simulink model "FaceDet_x4"  (Simulink 7.7)
settings: Solver=FixedStepDiscrete  StartTime=0  StopTime=10  RelTol=1e-3
libraries: simulink x257
(part 1 of 5)
settings Model: Creator=Ilia  LastModifiedBy=iliav
settings OptimizationCC: BlockReduction=off  ConditionallyExecuteInputs=off
settings DebuggingCC: StrictBusMsg=Warning

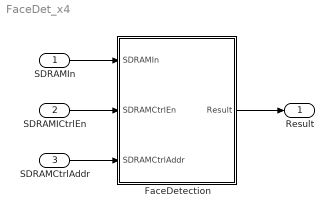
== system FaceDet_x4 ==
  SDRAMIn : Inport  OutDataTypeStr=uint(5)
  SDRAMICtrlEn : Inport  Port=2  OutDataTypeStr=boolean
  SDRAMCtrlAddr : Inport  Port=3  OutDataTypeStr=uint(12)
  FaceDetection : Subsystem
  Result : Outport
  wires:
  FaceDetection/1(Result) -> Result/1
  SDRAMIn/1 -> FaceDetection/1(SDRAMIn)
  SDRAMICtrlEn/1 -> FaceDetection/2(SDRAMCtrlEn)
  SDRAMCtrlAddr/1 -> FaceDetection/3(SDRAMCtrlAddr)

== system FaceDet_x4/FaceDetection ==
  SDRAMIn : Inport
  SDRAMCtrlEn : Inport  Port=2
  SDRAMCtrlAddr : Inport  Port=3
  DU : Subsystem
      mask Display: disp( 'Delay Lines\nUnit\n' )
  FU : Subsystem
      mask Display: disp( 'Face Detection\nUnit' )
  Result : Outport
  wires:
  DU/1(DOut24x5) -> FU/1(DIn24x5)
  SDRAMIn/1 -> DU/3(Data)
  SDRAMCtrlEn/1 -> DU/2(DLCtrlEn)
  SDRAMCtrlAddr/1 -> DU/1(DLCtrlAdr)
  FU/1(Result) -> Result/1

== system FaceDet_x4/FaceDetection/DU ==
  DLCtrlAdr : Inport
  DLCtrlEn : Inport  Port=2
  Data : Inport  Port=3
  Comb24DL : Mux  Inputs=3
  SplittedDL1 : Subsystem  TreatAsAtomicUnit=on
      mask Display: disp( 'Splitted DL\n8x512x5' )
  SplittedDL2 : Subsystem  TreatAsAtomicUnit=on
      mask Display: disp( 'Splitted DL\n8x512x5' )
  SplittedDL3 : Subsystem  TreatAsAtomicUnit=on
      mask Display: disp( 'Splitted DL\n8x512x5' )
  DOut24x5 : Outport
  wires:
  DLCtrlAdr/1 -> SplittedDL2/1(WrAdr), SplittedDL1/1(WrAdr), SplittedDL3/1(WrAdr), SplittedDL2/2(RdAdr), SplittedDL1/2(RdAdr), SplittedDL3/2(RdAdr)
  Comb24DL/1 -> DOut24x5/1
  SplittedDL3/1(DOut8x5) -> Comb24DL/1
  SplittedDL1/1(DOut8x5) -> Comb24DL/3
  SplittedDL2/1(DOut8x5) -> Comb24DL/2
  DLCtrlEn/1 -> SplittedDL2/3(WrEn), SplittedDL1/3(WrEn), SplittedDL3/3(WrEn)
  Data/1 -> SplittedDL3/4(DIn1x5), SplittedDL2/4(DIn1x5), SplittedDL1/4(DIn1x5)

== system FaceDet_x4/FaceDetection/FU ==
  DIn24x5 : Inport
  AccumulateAllFeatures : Subsystem  TreatAsAtomicUnit=on  mask(Accumulator){NBits=18}
      mask prompts: NBits "Number of Bits"
      mask help:
      | Accumulates incoming data. On reset only the state is initialized, meaning that when the reset is asserted the first valid output will be available from the next clock.
      | It is user responsiblity not to overcome the capacity of the accumulator.
      mask Help: web( ['E:\Ilia\Sightic\MakeVerilog\AccBlk\', 'AccBlkHelp.htm'] )
      mask Display: disp( 'Acc Blk\nBDelay = 0' )
  AddAllFeatures : Sum  Inputs=++++  OutDataTypeStr=uint(18)
  CalcIntegralImg : Subsystem  RequirementInfo={} %GIDa_13edc57c_8db7_4be7_a667_2f88c1a358e2  TreatAsAtomicUnit=on
  CalcNNVariance : Subsystem  TreatAsAtomicUnit=on
  CompToStrongTresh : RelationalOperator  Operator=<  OutDataTypeStr=boolean
  Demux1 : Demux
  Demux2 : Demux
  FaceDetectionControl : Stateflow chart  TreatAsAtomicUnit=on
      settings: RTWSystemCode=Inline
  FeatureCalcMachine0 : Subsystem  TreatAsAtomicUnit=on
      mask Display: disp( 'BDelay = \n' )
  FeatureCalcMachine1 : Subsystem  TreatAsAtomicUnit=on
      mask Display: disp( 'BDelay = \n' )
  FeatureCalcMachine2 : Subsystem  TreatAsAtomicUnit=on
      mask Display: disp( 'BDelay = \n' )
  FeatureCalcMachine3 : Subsystem  TreatAsAtomicUnit=on
      mask Display: disp( 'BDelay = \n' )
  MemBank : Subsystem
      mask Display: disp( '            Memory Block\n\n' )
  ValidNNTerm : Terminator
  Result : Outport
  wires:
  DIn24x5/1 -> CalcIntegralImg/1(DIn24x5), CalcNNVariance/2(Lines24x15)
  CalcIntegralImg/3(DOut24x15) -> FeatureCalcMachine2/2(Lines24x15), FeatureCalcMachine3/2(Lines24x15), FeatureCalcMachine1/2(Lines24x15), FeatureCalcMachine0/2(Lines24x15)
  MemBank/1(LineIdxs) -> FeatureCalcMachine2/3(LineIdxs), FeatureCalcMachine3/3(LineIdxs), FeatureCalcMachine1/3(LineIdxs), FeatureCalcMachine0/3(LineIdxs)
  MemBank/2(NodeWeights) -> FeatureCalcMachine2/4(NodeWeights), FeatureCalcMachine3/4(NodeWeights), FeatureCalcMachine1/4(NodeWeights), FeatureCalcMachine0/4(NodeWeights)
  FeatureCalcMachine0/1(FinalFeatureWeight) -> AddAllFeatures/1
  MemBank/4(StrongTresh) -> CompToStrongTresh/1
  CompToStrongTresh/1 -> Result/1
  AddAllFeatures/1 -> AccumulateAllFeatures/1(In)
  MemBank/3(FeatureData) -> Demux1/1
  Demux1/1 -> FeatureCalcMachine0/5(FeatureData)
  MemBank/5(WeakTresh) -> Demux2/1
  Demux2/1 -> FeatureCalcMachine0/6(WeakTresh)
  FeatureCalcMachine1/1(FinalFeatureWeight) -> AddAllFeatures/2
  FeatureCalcMachine2/1(FinalFeatureWeight) -> AddAllFeatures/3
  Demux1/2 -> FeatureCalcMachine1/5(FeatureData)
  AccumulateAllFeatures/1(Acc) -> CompToStrongTresh/2
  Demux1/3 -> FeatureCalcMachine2/5(FeatureData)
  Demux2/2 -> FeatureCalcMachine1/6(WeakTresh)
  Demux2/3 -> FeatureCalcMachine2/6(WeakTresh)
  FeatureCalcMachine3/1(FinalFeatureWeight) -> AddAllFeatures/4
  Demux1/4 -> FeatureCalcMachine3/5(FeatureData)
  Demux2/4 -> FeatureCalcMachine3/6(WeakTresh)
  CalcNNVariance/1(SqVar) -> FeatureCalcMachine2/1(SqVar), FeatureCalcMachine3/1(SqVar), FeatureCalcMachine1/1(SqVar), FeatureCalcMachine0/1(SqVar)
  CalcIntegralImg/1(MeanBlkVal) -> CalcNNVariance/3(MeanBlkVal)
  CalcIntegralImg/2(ValidNN) -> ValidNNTerm/1
  FaceDetectionControl/3(LatchIdxLatch) -> MemBank/1(LineIdxsLatch)
  FaceDetectionControl/4(LatchIdxExt) -> MemBank/2(LineIdxsExt)
  FaceDetectionControl/5(NodeWeightsCtrlRdAdr) -> MemBank/3(NodeWeightsCtrlRdAdr)
  FaceDetectionControl/6(NodeWeightsCtrlWrAdr) -> MemBank/4(NodeWeightsCtrlWrAdr)
  FaceDetectionControl/7(NodeWeightsCtrlEn) -> MemBank/5(NodeWeightsCtrlEn)
  FaceDetectionControl/8(NodeWeightsExt) -> MemBank/6(NodeWeightsExt)
  FaceDetectionControl/9(FeatureDataLatch) -> MemBank/7(FeatureDataLatch)
  FaceDetectionControl/10(FeatureDataExt) -> MemBank/8(FeatureDataExt)
  FaceDetectionControl/11(WeakTreshLatch) -> MemBank/9(WeakTreshLatch)
  FaceDetectionControl/12(WeakTreshExt) -> MemBank/10(WeakTreshExt)
  FaceDetectionControl/13(StrongTreshLatch) -> MemBank/11(StrongTreshLatch)
  FaceDetectionControl/14(StrongTreshExt) -> MemBank/12(StrongTreshExt)
  FaceDetectionControl/2(Rst) -> CalcIntegralImg/2(Rst), CalcNNVariance/1(Rst), AccumulateAllFeatures/3(Rst)
  FaceDetectionControl/1(En) -> CalcIntegralImg/3(En), AccumulateAllFeatures/2(En)

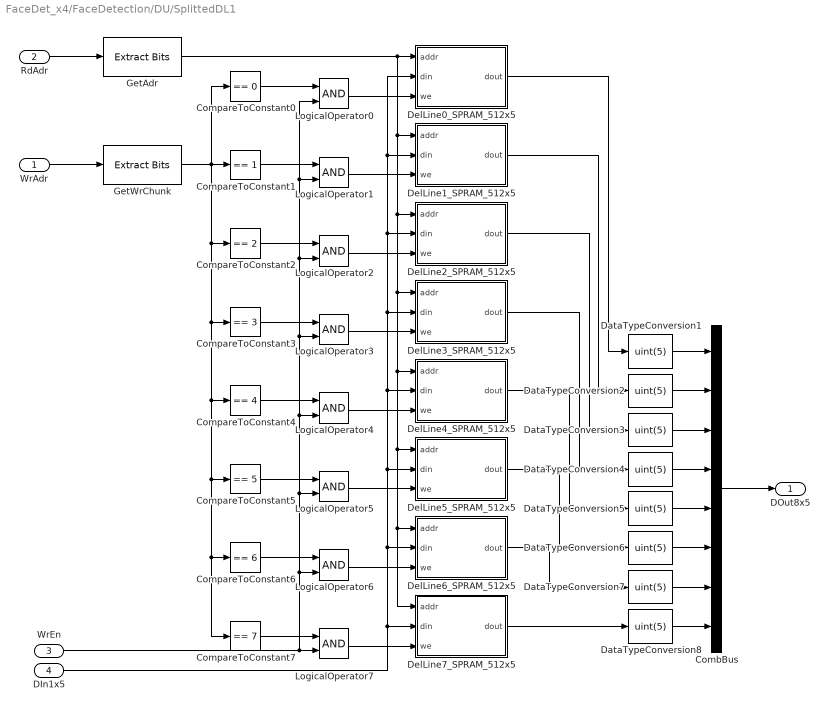
== system FaceDet_x4/FaceDetection/DU/SplittedDL1 ==
  WrAdr : Inport
  RdAdr : Inport  Port=2
  WrEn : Inport  Port=3
  DIn1x5 : Inport  Port=4
  CombBus : Mux  Inputs=8
  CompareToConstant0 : simulink/Logic and Bit Operations/Compare To Constant  SystemSampleTime=-1  relop===  const=0  LogicOutDataTypeMode=boolean  ZeroCross=off
  CompareToConstant1 : simulink/Logic and Bit Operations/Compare To Constant  SystemSampleTime=-1  relop===  const=1  LogicOutDataTypeMode=boolean  ZeroCross=off
  CompareToConstant2 : simulink/Logic and Bit Operations/Compare To Constant  SystemSampleTime=-1  relop===  const=2  LogicOutDataTypeMode=boolean  ZeroCross=off
  CompareToConstant3 : simulink/Logic and Bit Operations/Compare To Constant  SystemSampleTime=-1  relop===  const=3  LogicOutDataTypeMode=boolean  ZeroCross=off
  CompareToConstant4 : simulink/Logic and Bit Operations/Compare To Constant  SystemSampleTime=-1  relop===  const=4  LogicOutDataTypeMode=boolean  ZeroCross=off
  CompareToConstant5 : simulink/Logic and Bit Operations/Compare To Constant  SystemSampleTime=-1  relop===  const=5  LogicOutDataTypeMode=boolean  ZeroCross=off
  CompareToConstant6 : simulink/Logic and Bit Operations/Compare To Constant  SystemSampleTime=-1  relop===  const=6  LogicOutDataTypeMode=boolean  ZeroCross=off
  CompareToConstant7 : simulink/Logic and Bit Operations/Compare To Constant  SystemSampleTime=-1  relop===  const=7  LogicOutDataTypeMode=boolean  ZeroCross=off
  DataTypeConversion{1..8} (8 alike) : DataTypeConversion  OutDataTypeStr=uint(5)
  DelLine0_SPRAM_512x5 : Subsystem  TreatAsAtomicUnit=on  mask(Single-port RAM){BlkNamePrefix='DelLine0', depth_bits=9, width_bits=5, dout_type=New data}
      mask prompts: BlkNamePrefix "Block name prefix:"; depth_bits "Address port width (2 to 16):"; width_bits "Data port width:"; dout_type "Output data during write:"
      mask help:
      | This block simulates a single-port RAM (based on hdllib).
      |
      | The address port width is limited to between 2 to 16 bits.
      mask init:
      | dout_type = 1;
      | 
      | if (isempty(depth_bits) || isempty(width_bits))
      |     set_param(gcb, 'Name', 'Single Port RAM');
      | else
      |     
      |     ram_elements = 2^depth_bits;
      |     
      |     NewName = ['SPRAM_', int2str(ram_elements), ...
      |         'x', int2str(width_bits)];
      |     
      |     if ~isempty(BlkNamePrefix)
      |         NewName = [BlkNamePrefix, '_', NewName];
      |     end
      |     
      |     set_param(gcb, 'Name', NewName);
      | 
      | end
      mask StyleString: edit,edit,edit,popup(New data|Old data)
      mask Display: color('gray'); text(.5, .05, '{\fontsize{6}BRCM}', 'texmode', 'on', 'verticalAlignment', 'bottom', 'horizontalAlignment', 'center');
  DelLine1_SPRAM_512x5 : Subsystem  TreatAsAtomicUnit=on  mask(Single-port RAM){BlkNamePrefix='DelLine1', depth_bits=9, width_bits=5, dout_type=New data}
      mask prompts: BlkNamePrefix "Block name prefix:"; depth_bits "Address port width (2 to 16):"; width_bits "Data port width:"; dout_type "Output data during write:"
      mask help:
      | This block simulates a single-port RAM (based on hdllib).
      |
      | The address port width is limited to between 2 to 16 bits.
      mask init: same as FaceDet_x4/FaceDetection/DU/SplittedDL1/DelLine0_SPRAM_512x5
      mask StyleString: edit,edit,edit,popup(New data|Old data)
      mask Display: color('gray'); text(.5, .05, '{\fontsize{6}BRCM}', 'texmode', 'on', 'verticalAlignment', 'bottom', 'horizontalAlignment', 'center');
  DelLine2_SPRAM_512x5 : Subsystem  TreatAsAtomicUnit=on  mask(Single-port RAM){BlkNamePrefix='DelLine2', depth_bits=9, width_bits=5, dout_type=New data}
      mask prompts: BlkNamePrefix "Block name prefix:"; depth_bits "Address port width (2 to 16):"; width_bits "Data port width:"; dout_type "Output data during write:"
      mask help:
      | This block simulates a single-port RAM (based on hdllib).
      |
      | The address port width is limited to between 2 to 16 bits.
      mask init: same as FaceDet_x4/FaceDetection/DU/SplittedDL1/DelLine0_SPRAM_512x5
      mask StyleString: edit,edit,edit,popup(New data|Old data)
      mask Display: color('gray'); text(.5, .05, '{\fontsize{6}BRCM}', 'texmode', 'on', 'verticalAlignment', 'bottom', 'horizontalAlignment', 'center');
  DelLine3_SPRAM_512x5 : Subsystem  TreatAsAtomicUnit=on  mask(Single-port RAM){BlkNamePrefix='DelLine3', depth_bits=9, width_bits=5, dout_type=New data}
      mask prompts: BlkNamePrefix "Block name prefix:"; depth_bits "Address port width (2 to 16):"; width_bits "Data port width:"; dout_type "Output data during write:"
      mask help:
      | This block simulates a single-port RAM (based on hdllib).
      |
      | The address port width is limited to between 2 to 16 bits.
      mask init: same as FaceDet_x4/FaceDetection/DU/SplittedDL1/DelLine0_SPRAM_512x5
      mask StyleString: edit,edit,edit,popup(New data|Old data)
      mask Display: color('gray'); text(.5, .05, '{\fontsize{6}BRCM}', 'texmode', 'on', 'verticalAlignment', 'bottom', 'horizontalAlignment', 'center');
  DelLine4_SPRAM_512x5 : Subsystem  TreatAsAtomicUnit=on  mask(Single-port RAM){BlkNamePrefix='DelLine4', depth_bits=9, width_bits=5, dout_type=New data}
      mask prompts: BlkNamePrefix "Block name prefix:"; depth_bits "Address port width (2 to 16):"; width_bits "Data port width:"; dout_type "Output data during write:"
      mask help:
      | This block simulates a single-port RAM (based on hdllib).
      |
      | The address port width is limited to between 2 to 16 bits.
      mask init: same as FaceDet_x4/FaceDetection/DU/SplittedDL1/DelLine0_SPRAM_512x5
      mask StyleString: edit,edit,edit,popup(New data|Old data)
      mask Display: color('gray'); text(.5, .05, '{\fontsize{6}BRCM}', 'texmode', 'on', 'verticalAlignment', 'bottom', 'horizontalAlignment', 'center');
  DelLine5_SPRAM_512x5 : Subsystem  TreatAsAtomicUnit=on  mask(Single-port RAM){BlkNamePrefix='DelLine5', depth_bits=9, width_bits=5, dout_type=New data}
      mask prompts: BlkNamePrefix "Block name prefix:"; depth_bits "Address port width (2 to 16):"; width_bits "Data port width:"; dout_type "Output data during write:"
      mask help:
      | This block simulates a single-port RAM (based on hdllib).
      |
      | The address port width is limited to between 2 to 16 bits.
      mask init: same as FaceDet_x4/FaceDetection/DU/SplittedDL1/DelLine0_SPRAM_512x5
      mask StyleString: edit,edit,edit,popup(New data|Old data)
      mask Display: color('gray'); text(.5, .05, '{\fontsize{6}BRCM}', 'texmode', 'on', 'verticalAlignment', 'bottom', 'horizontalAlignment', 'center');
  DelLine6_SPRAM_512x5 : Subsystem  TreatAsAtomicUnit=on  mask(Single-port RAM){BlkNamePrefix='DelLine6', depth_bits=9, width_bits=5, dout_type=New data}
      mask prompts: BlkNamePrefix "Block name prefix:"; depth_bits "Address port width (2 to 16):"; width_bits "Data port width:"; dout_type "Output data during write:"
      mask help:
      | This block simulates a single-port RAM (based on hdllib).
      |
      | The address port width is limited to between 2 to 16 bits.
      mask init: same as FaceDet_x4/FaceDetection/DU/SplittedDL1/DelLine0_SPRAM_512x5
      mask StyleString: edit,edit,edit,popup(New data|Old data)
      mask Display: color('gray'); text(.5, .05, '{\fontsize{6}BRCM}', 'texmode', 'on', 'verticalAlignment', 'bottom', 'horizontalAlignment', 'center');
  DelLine7_SPRAM_512x5 : Subsystem  TreatAsAtomicUnit=on  mask(Single-port RAM){BlkNamePrefix='DelLine7', depth_bits=9, width_bits=5, dout_type=New data}
      mask prompts: BlkNamePrefix "Block name prefix:"; depth_bits "Address port width (2 to 16):"; width_bits "Data port width:"; dout_type "Output data during write:"
      mask help:
      | This block simulates a single-port RAM (based on hdllib).
      |
      | The address port width is limited to between 2 to 16 bits.
      mask init: same as FaceDet_x4/FaceDetection/DU/SplittedDL1/DelLine0_SPRAM_512x5
      mask StyleString: edit,edit,edit,popup(New data|Old data)
      mask Display: color('gray'); text(.5, .05, '{\fontsize{6}BRCM}', 'texmode', 'on', 'verticalAlignment', 'bottom', 'horizontalAlignment', 'center');
  GetAdr : simulink/Logic and Bit Operations/Extract Bits  SystemSampleTime=-1  bitsToExtract=Range of bits  numBits=8  bitIdxRange=[0 8]  outScalingMode=Treat bit field as an integer
  GetWrChunk : simulink/Logic and Bit Operations/Extract Bits  SystemSampleTime=-1  bitsToExtract=Range of bits  numBits=8  bitIdxRange=[9 11]  outScalingMode=Treat bit field as an integer
  LogicalOperator{0..7} (8 alike) : Logic  AllPortsSameDT=off  OutDataTypeStr=boolean
  DOut8x5 : Outport
  wires:
  CompareToConstant7/1 -> LogicalOperator7/1
  CompareToConstant6/1 -> LogicalOperator6/1
  CompareToConstant5/1 -> LogicalOperator5/1
  CompareToConstant4/1 -> LogicalOperator4/1
  CompareToConstant3/1 -> LogicalOperator3/1
  CompareToConstant2/1 -> LogicalOperator2/1
  CompareToConstant1/1 -> LogicalOperator1/1
  GetWrChunk/1 -> CompareToConstant7/1, CompareToConstant6/1, CompareToConstant5/1, CompareToConstant4/1, CompareToConstant3/1, CompareToConstant2/1, CompareToConstant1/1, CompareToConstant0/1
  CompareToConstant0/1 -> LogicalOperator0/1
  WrEn/1 -> LogicalOperator0/2, LogicalOperator1/2, LogicalOperator2/2, LogicalOperator3/2, LogicalOperator4/2, LogicalOperator5/2, LogicalOperator6/2, LogicalOperator7/2
  LogicalOperator7/1 -> DelLine7_SPRAM_512x5/3(we)
  LogicalOperator6/1 -> DelLine6_SPRAM_512x5/3(we)
  LogicalOperator5/1 -> DelLine5_SPRAM_512x5/3(we)
  LogicalOperator4/1 -> DelLine4_SPRAM_512x5/3(we)
  LogicalOperator3/1 -> DelLine3_SPRAM_512x5/3(we)
  DIn1x5/1 -> DelLine7_SPRAM_512x5/2(din), DelLine6_SPRAM_512x5/2(din), DelLine5_SPRAM_512x5/2(din), DelLine4_SPRAM_512x5/2(din), DelLine3_SPRAM_512x5/2(din), DelLine2_SPRAM_512x5/2(din), DelLine0_SPRAM_512x5/2(din), DelLine1_SPRAM_512x5/2(din)
  LogicalOperator2/1 -> DelLine2_SPRAM_512x5/3(we)
  LogicalOperator0/1 -> DelLine0_SPRAM_512x5/3(we)
  LogicalOperator1/1 -> DelLine1_SPRAM_512x5/3(we)
  WrAdr/1 -> GetWrChunk/1
  GetAdr/1 -> DelLine0_SPRAM_512x5/1(addr), DelLine2_SPRAM_512x5/1(addr), DelLine3_SPRAM_512x5/1(addr), DelLine4_SPRAM_512x5/1(addr), DelLine5_SPRAM_512x5/1(addr), DelLine7_SPRAM_512x5/1(addr), DelLine6_SPRAM_512x5/1(addr), DelLine1_SPRAM_512x5/1(addr)
  DataTypeConversion8/1 -> CombBus/8
  DataTypeConversion7/1 -> CombBus/7
  DataTypeConversion6/1 -> CombBus/6
  DataTypeConversion5/1 -> CombBus/5
  DataTypeConversion4/1 -> CombBus/4
  DataTypeConversion3/1 -> CombBus/3
  DataTypeConversion2/1 -> CombBus/2
  DataTypeConversion1/1 -> CombBus/1
  DelLine7_SPRAM_512x5/1(dout) -> DataTypeConversion8/1
  DelLine6_SPRAM_512x5/1(dout) -> DataTypeConversion7/1
  DelLine5_SPRAM_512x5/1(dout) -> DataTypeConversion6/1
  DelLine4_SPRAM_512x5/1(dout) -> DataTypeConversion5/1
  DelLine3_SPRAM_512x5/1(dout) -> DataTypeConversion4/1
  DelLine2_SPRAM_512x5/1(dout) -> DataTypeConversion3/1
  DelLine1_SPRAM_512x5/1(dout) -> DataTypeConversion2/1
  CombBus/1 -> DOut8x5/1
  RdAdr/1 -> GetAdr/1
  DelLine0_SPRAM_512x5/1(dout) -> DataTypeConversion1/1

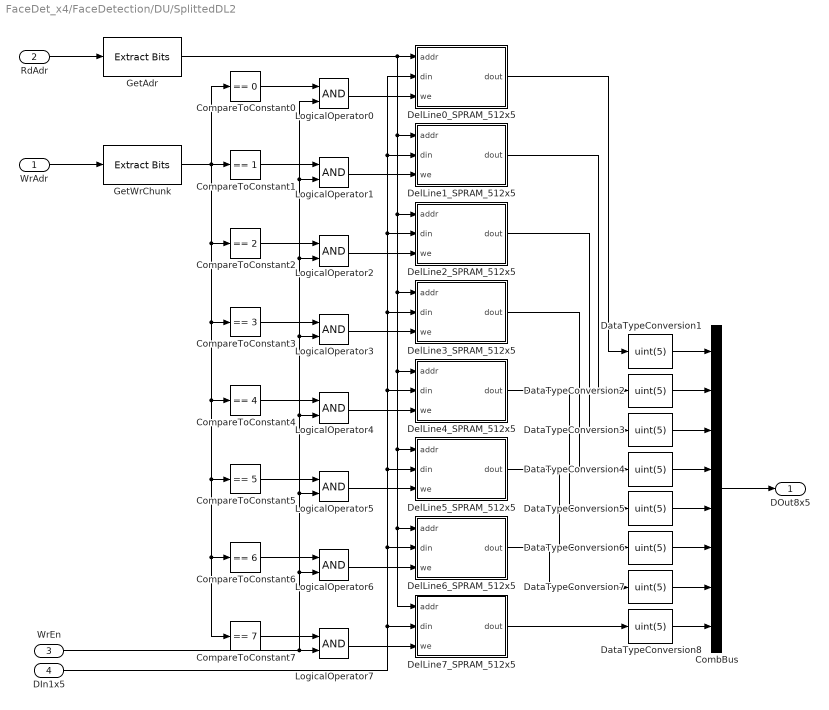
== system FaceDet_x4/FaceDetection/DU/SplittedDL2 ==
  WrAdr : Inport
  RdAdr : Inport  Port=2
  WrEn : Inport  Port=3
  DIn1x5 : Inport  Port=4
  CombBus : Mux  Inputs=8
  CompareToConstant0 : simulink/Logic and Bit Operations/Compare To Constant  SystemSampleTime=-1  relop===  const=0  LogicOutDataTypeMode=boolean  ZeroCross=off
  CompareToConstant1 : simulink/Logic and Bit Operations/Compare To Constant  SystemSampleTime=-1  relop===  const=1  LogicOutDataTypeMode=boolean  ZeroCross=off
  CompareToConstant2 : simulink/Logic and Bit Operations/Compare To Constant  SystemSampleTime=-1  relop===  const=2  LogicOutDataTypeMode=boolean  ZeroCross=off
  CompareToConstant3 : simulink/Logic and Bit Operations/Compare To Constant  SystemSampleTime=-1  relop===  const=3  LogicOutDataTypeMode=boolean  ZeroCross=off
  CompareToConstant4 : simulink/Logic and Bit Operations/Compare To Constant  SystemSampleTime=-1  relop===  const=4  LogicOutDataTypeMode=boolean  ZeroCross=off
  CompareToConstant5 : simulink/Logic and Bit Operations/Compare To Constant  SystemSampleTime=-1  relop===  const=5  LogicOutDataTypeMode=boolean  ZeroCross=off
  CompareToConstant6 : simulink/Logic and Bit Operations/Compare To Constant  SystemSampleTime=-1  relop===  const=6  LogicOutDataTypeMode=boolean  ZeroCross=off
  CompareToConstant7 : simulink/Logic and Bit Operations/Compare To Constant  SystemSampleTime=-1  relop===  const=7  LogicOutDataTypeMode=boolean  ZeroCross=off
  DataTypeConversion{1..8} (8 alike) : DataTypeConversion  OutDataTypeStr=uint(5)
  DelLine0_SPRAM_512x5 : Subsystem  TreatAsAtomicUnit=on  mask(Single-port RAM){BlkNamePrefix='DelLine0', depth_bits=9, width_bits=5, dout_type=New data}
      mask prompts: BlkNamePrefix "Block name prefix:"; depth_bits "Address port width (2 to 16):"; width_bits "Data port width:"; dout_type "Output data during write:"
      mask help:
      | This block simulates a single-port RAM (based on hdllib).
      |
      | The address port width is limited to between 2 to 16 bits.
      mask init: same as FaceDet_x4/FaceDetection/DU/SplittedDL1/DelLine0_SPRAM_512x5
      mask StyleString: edit,edit,edit,popup(New data|Old data)
      mask Display: color('gray'); text(.5, .05, '{\fontsize{6}BRCM}', 'texmode', 'on', 'verticalAlignment', 'bottom', 'horizontalAlignment', 'center');
  DelLine1_SPRAM_512x5 : Subsystem  TreatAsAtomicUnit=on  mask(Single-port RAM){BlkNamePrefix='DelLine1', depth_bits=9, width_bits=5, dout_type=New data}
      mask prompts: BlkNamePrefix "Block name prefix:"; depth_bits "Address port width (2 to 16):"; width_bits "Data port width:"; dout_type "Output data during write:"
      mask help:
      | This block simulates a single-port RAM (based on hdllib).
      |
      | The address port width is limited to between 2 to 16 bits.
      mask init: same as FaceDet_x4/FaceDetection/DU/SplittedDL1/DelLine0_SPRAM_512x5
      mask StyleString: edit,edit,edit,popup(New data|Old data)
      mask Display: color('gray'); text(.5, .05, '{\fontsize{6}BRCM}', 'texmode', 'on', 'verticalAlignment', 'bottom', 'horizontalAlignment', 'center');
  DelLine2_SPRAM_512x5 : Subsystem  TreatAsAtomicUnit=on  mask(Single-port RAM){BlkNamePrefix='DelLine2', depth_bits=9, width_bits=5, dout_type=New data}
      mask prompts: BlkNamePrefix "Block name prefix:"; depth_bits "Address port width (2 to 16):"; width_bits "Data port width:"; dout_type "Output data during write:"
      mask help:
      | This block simulates a single-port RAM (based on hdllib).
      |
      | The address port width is limited to between 2 to 16 bits.
      mask init: same as FaceDet_x4/FaceDetection/DU/SplittedDL1/DelLine0_SPRAM_512x5
      mask StyleString: edit,edit,edit,popup(New data|Old data)
      mask Display: color('gray'); text(.5, .05, '{\fontsize{6}BRCM}', 'texmode', 'on', 'verticalAlignment', 'bottom', 'horizontalAlignment', 'center');
  DelLine3_SPRAM_512x5 : Subsystem  TreatAsAtomicUnit=on  mask(Single-port RAM){BlkNamePrefix='DelLine3', depth_bits=9, width_bits=5, dout_type=New data}
      mask prompts: BlkNamePrefix "Block name prefix:"; depth_bits "Address port width (2 to 16):"; width_bits "Data port width:"; dout_type "Output data during write:"
      mask help:
      | This block simulates a single-port RAM (based on hdllib).
      |
      | The address port width is limited to between 2 to 16 bits.
      mask init: same as FaceDet_x4/FaceDetection/DU/SplittedDL1/DelLine0_SPRAM_512x5
      mask StyleString: edit,edit,edit,popup(New data|Old data)
      mask Display: color('gray'); text(.5, .05, '{\fontsize{6}BRCM}', 'texmode', 'on', 'verticalAlignment', 'bottom', 'horizontalAlignment', 'center');
  DelLine4_SPRAM_512x5 : Subsystem  TreatAsAtomicUnit=on  mask(Single-port RAM){BlkNamePrefix='DelLine4', depth_bits=9, width_bits=5, dout_type=New data}
      mask prompts: BlkNamePrefix "Block name prefix:"; depth_bits "Address port width (2 to 16):"; width_bits "Data port width:"; dout_type "Output data during write:"
      mask help:
      | This block simulates a single-port RAM (based on hdllib).
      |
      | The address port width is limited to between 2 to 16 bits.
      mask init: same as FaceDet_x4/FaceDetection/DU/SplittedDL1/DelLine0_SPRAM_512x5
      mask StyleString: edit,edit,edit,popup(New data|Old data)
      mask Display: color('gray'); text(.5, .05, '{\fontsize{6}BRCM}', 'texmode', 'on', 'verticalAlignment', 'bottom', 'horizontalAlignment', 'center');
  DelLine5_SPRAM_512x5 : Subsystem  TreatAsAtomicUnit=on  mask(Single-port RAM){BlkNamePrefix='DelLine5', depth_bits=9, width_bits=5, dout_type=New data}
      mask prompts: BlkNamePrefix "Block name prefix:"; depth_bits "Address port width (2 to 16):"; width_bits "Data port width:"; dout_type "Output data during write:"
      mask help:
      | This block simulates a single-port RAM (based on hdllib).
      |
      | The address port width is limited to between 2 to 16 bits.
      mask init: same as FaceDet_x4/FaceDetection/DU/SplittedDL1/DelLine0_SPRAM_512x5
      mask StyleString: edit,edit,edit,popup(New data|Old data)
      mask Display: color('gray'); text(.5, .05, '{\fontsize{6}BRCM}', 'texmode', 'on', 'verticalAlignment', 'bottom', 'horizontalAlignment', 'center');
  DelLine6_SPRAM_512x5 : Subsystem  TreatAsAtomicUnit=on  mask(Single-port RAM){BlkNamePrefix='DelLine6', depth_bits=9, width_bits=5, dout_type=New data}
      mask prompts: BlkNamePrefix "Block name prefix:"; depth_bits "Address port width (2 to 16):"; width_bits "Data port width:"; dout_type "Output data during write:"
      mask help:
      | This block simulates a single-port RAM (based on hdllib).
      |
      | The address port width is limited to between 2 to 16 bits.
      mask init: same as FaceDet_x4/FaceDetection/DU/SplittedDL1/DelLine0_SPRAM_512x5
      mask StyleString: edit,edit,edit,popup(New data|Old data)
      mask Display: color('gray'); text(.5, .05, '{\fontsize{6}BRCM}', 'texmode', 'on', 'verticalAlignment', 'bottom', 'horizontalAlignment', 'center');
  DelLine7_SPRAM_512x5 : Subsystem  TreatAsAtomicUnit=on  mask(Single-port RAM){BlkNamePrefix='DelLine7', depth_bits=9, width_bits=5, dout_type=New data}
      mask prompts: BlkNamePrefix "Block name prefix:"; depth_bits "Address port width (2 to 16):"; width_bits "Data port width:"; dout_type "Output data during write:"
      mask help:
      | This block simulates a single-port RAM (based on hdllib).
      |
      | The address port width is limited to between 2 to 16 bits.
      mask init: same as FaceDet_x4/FaceDetection/DU/SplittedDL1/DelLine0_SPRAM_512x5
      mask StyleString: edit,edit,edit,popup(New data|Old data)
      mask Display: color('gray'); text(.5, .05, '{\fontsize{6}BRCM}', 'texmode', 'on', 'verticalAlignment', 'bottom', 'horizontalAlignment', 'center');
  GetAdr : simulink/Logic and Bit Operations/Extract Bits  SystemSampleTime=-1  bitsToExtract=Range of bits  numBits=8  bitIdxRange=[0 8]  outScalingMode=Treat bit field as an integer
  GetWrChunk : simulink/Logic and Bit Operations/Extract Bits  SystemSampleTime=-1  bitsToExtract=Range of bits  numBits=8  bitIdxRange=[9 11]  outScalingMode=Treat bit field as an integer
  LogicalOperator{0..7} (8 alike) : Logic  AllPortsSameDT=off  OutDataTypeStr=boolean
  DOut8x5 : Outport
  wires:
  DelLine0_SPRAM_512x5/1(dout) -> DataTypeConversion1/1
  RdAdr/1 -> GetAdr/1
  CombBus/1 -> DOut8x5/1
  DelLine1_SPRAM_512x5/1(dout) -> DataTypeConversion2/1
  DelLine2_SPRAM_512x5/1(dout) -> DataTypeConversion3/1
  DelLine3_SPRAM_512x5/1(dout) -> DataTypeConversion4/1
  DelLine4_SPRAM_512x5/1(dout) -> DataTypeConversion5/1
  DelLine5_SPRAM_512x5/1(dout) -> DataTypeConversion6/1
  DelLine6_SPRAM_512x5/1(dout) -> DataTypeConversion7/1
  DelLine7_SPRAM_512x5/1(dout) -> DataTypeConversion8/1
  DataTypeConversion1/1 -> CombBus/1
  DataTypeConversion2/1 -> CombBus/2
  DataTypeConversion3/1 -> CombBus/3
  DataTypeConversion4/1 -> CombBus/4
  DataTypeConversion5/1 -> CombBus/5
  DataTypeConversion6/1 -> CombBus/6
  DataTypeConversion7/1 -> CombBus/7
  DataTypeConversion8/1 -> CombBus/8
  GetAdr/1 -> DelLine1_SPRAM_512x5/1(addr), DelLine6_SPRAM_512x5/1(addr), DelLine7_SPRAM_512x5/1(addr), DelLine5_SPRAM_512x5/1(addr), DelLine4_SPRAM_512x5/1(addr), DelLine3_SPRAM_512x5/1(addr), DelLine2_SPRAM_512x5/1(addr), DelLine0_SPRAM_512x5/1(addr)
  WrAdr/1 -> GetWrChunk/1
  LogicalOperator1/1 -> DelLine1_SPRAM_512x5/3(we)
  LogicalOperator0/1 -> DelLine0_SPRAM_512x5/3(we)
  LogicalOperator2/1 -> DelLine2_SPRAM_512x5/3(we)
  DIn1x5/1 -> DelLine1_SPRAM_512x5/2(din), DelLine0_SPRAM_512x5/2(din), DelLine2_SPRAM_512x5/2(din), DelLine3_SPRAM_512x5/2(din), DelLine4_SPRAM_512x5/2(din), DelLine5_SPRAM_512x5/2(din), DelLine6_SPRAM_512x5/2(din), DelLine7_SPRAM_512x5/2(din)
  LogicalOperator3/1 -> DelLine3_SPRAM_512x5/3(we)
  LogicalOperator4/1 -> DelLine4_SPRAM_512x5/3(we)
  LogicalOperator5/1 -> DelLine5_SPRAM_512x5/3(we)
  LogicalOperator6/1 -> DelLine6_SPRAM_512x5/3(we)
  LogicalOperator7/1 -> DelLine7_SPRAM_512x5/3(we)
  WrEn/1 -> LogicalOperator7/2, LogicalOperator6/2, LogicalOperator5/2, LogicalOperator4/2, LogicalOperator3/2, LogicalOperator2/2, LogicalOperator1/2, LogicalOperator0/2
  CompareToConstant0/1 -> LogicalOperator0/1
  GetWrChunk/1 -> CompareToConstant0/1, CompareToConstant1/1, CompareToConstant2/1, CompareToConstant3/1, CompareToConstant4/1, CompareToConstant5/1, CompareToConstant6/1, CompareToConstant7/1
  CompareToConstant1/1 -> LogicalOperator1/1
  CompareToConstant2/1 -> LogicalOperator2/1
  CompareToConstant3/1 -> LogicalOperator3/1
  CompareToConstant4/1 -> LogicalOperator4/1
  CompareToConstant5/1 -> LogicalOperator5/1
  CompareToConstant6/1 -> LogicalOperator6/1
  CompareToConstant7/1 -> LogicalOperator7/1

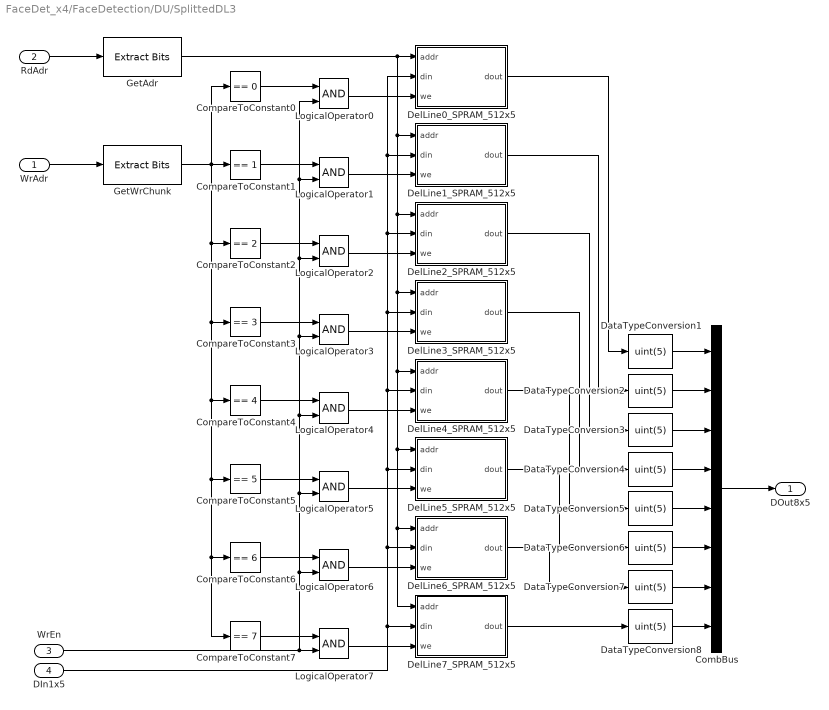
== system FaceDet_x4/FaceDetection/DU/SplittedDL3 ==
  WrAdr : Inport
  RdAdr : Inport  Port=2
  WrEn : Inport  Port=3
  DIn1x5 : Inport  Port=4
  CombBus : Mux  Inputs=8
  CompareToConstant0 : simulink/Logic and Bit Operations/Compare To Constant  SystemSampleTime=-1  relop===  const=0  LogicOutDataTypeMode=boolean  ZeroCross=off
  CompareToConstant1 : simulink/Logic and Bit Operations/Compare To Constant  SystemSampleTime=-1  relop===  const=1  LogicOutDataTypeMode=boolean  ZeroCross=off
  CompareToConstant2 : simulink/Logic and Bit Operations/Compare To Constant  SystemSampleTime=-1  relop===  const=2  LogicOutDataTypeMode=boolean  ZeroCross=off
  CompareToConstant3 : simulink/Logic and Bit Operations/Compare To Constant  SystemSampleTime=-1  relop===  const=3  LogicOutDataTypeMode=boolean  ZeroCross=off
  CompareToConstant4 : simulink/Logic and Bit Operations/Compare To Constant  SystemSampleTime=-1  relop===  const=4  LogicOutDataTypeMode=boolean  ZeroCross=off
  CompareToConstant5 : simulink/Logic and Bit Operations/Compare To Constant  SystemSampleTime=-1  relop===  const=5  LogicOutDataTypeMode=boolean  ZeroCross=off
  CompareToConstant6 : simulink/Logic and Bit Operations/Compare To Constant  SystemSampleTime=-1  relop===  const=6  LogicOutDataTypeMode=boolean  ZeroCross=off
  CompareToConstant7 : simulink/Logic and Bit Operations/Compare To Constant  SystemSampleTime=-1  relop===  const=7  LogicOutDataTypeMode=boolean  ZeroCross=off
  DataTypeConversion{1..8} (8 alike) : DataTypeConversion  OutDataTypeStr=uint(5)
  DelLine0_SPRAM_512x5 : Subsystem  TreatAsAtomicUnit=on  mask(Single-port RAM){BlkNamePrefix='DelLine0', depth_bits=9, width_bits=5, dout_type=New data}
      mask prompts: BlkNamePrefix "Block name prefix:"; depth_bits "Address port width (2 to 16):"; width_bits "Data port width:"; dout_type "Output data during write:"
      mask help:
      | This block simulates a single-port RAM (based on hdllib).
      |
      | The address port width is limited to between 2 to 16 bits.
      mask init: same as FaceDet_x4/FaceDetection/DU/SplittedDL1/DelLine0_SPRAM_512x5
      mask StyleString: edit,edit,edit,popup(New data|Old data)
      mask Display: color('gray'); text(.5, .05, '{\fontsize{6}BRCM}', 'texmode', 'on', 'verticalAlignment', 'bottom', 'horizontalAlignment', 'center');
  DelLine1_SPRAM_512x5 : Subsystem  TreatAsAtomicUnit=on  mask(Single-port RAM){BlkNamePrefix='DelLine1', depth_bits=9, width_bits=5, dout_type=New data}
      mask prompts: BlkNamePrefix "Block name prefix:"; depth_bits "Address port width (2 to 16):"; width_bits "Data port width:"; dout_type "Output data during write:"
      mask help:
      | This block simulates a single-port RAM (based on hdllib).
      |
      | The address port width is limited to between 2 to 16 bits.
      mask init: same as FaceDet_x4/FaceDetection/DU/SplittedDL1/DelLine0_SPRAM_512x5
      mask StyleString: edit,edit,edit,popup(New data|Old data)
      mask Display: color('gray'); text(.5, .05, '{\fontsize{6}BRCM}', 'texmode', 'on', 'verticalAlignment', 'bottom', 'horizontalAlignment', 'center');
  DelLine2_SPRAM_512x5 : Subsystem  TreatAsAtomicUnit=on  mask(Single-port RAM){BlkNamePrefix='DelLine2', depth_bits=9, width_bits=5, dout_type=New data}
      mask prompts: BlkNamePrefix "Block name prefix:"; depth_bits "Address port width (2 to 16):"; width_bits "Data port width:"; dout_type "Output data during write:"
      mask help:
      | This block simulates a single-port RAM (based on hdllib).
      |
      | The address port width is limited to between 2 to 16 bits.
      mask init: same as FaceDet_x4/FaceDetection/DU/SplittedDL1/DelLine0_SPRAM_512x5
      mask StyleString: edit,edit,edit,popup(New data|Old data)
      mask Display: color('gray'); text(.5, .05, '{\fontsize{6}BRCM}', 'texmode', 'on', 'verticalAlignment', 'bottom', 'horizontalAlignment', 'center');
  DelLine3_SPRAM_512x5 : Subsystem  TreatAsAtomicUnit=on  mask(Single-port RAM){BlkNamePrefix='DelLine3', depth_bits=9, width_bits=5, dout_type=New data}
      mask prompts: BlkNamePrefix "Block name prefix:"; depth_bits "Address port width (2 to 16):"; width_bits "Data port width:"; dout_type "Output data during write:"
      mask help:
      | This block simulates a single-port RAM (based on hdllib).
      |
      | The address port width is limited to between 2 to 16 bits.
      mask init: same as FaceDet_x4/FaceDetection/DU/SplittedDL1/DelLine0_SPRAM_512x5
      mask StyleString: edit,edit,edit,popup(New data|Old data)
      mask Display: color('gray'); text(.5, .05, '{\fontsize{6}BRCM}', 'texmode', 'on', 'verticalAlignment', 'bottom', 'horizontalAlignment', 'center');
  DelLine4_SPRAM_512x5 : Subsystem  TreatAsAtomicUnit=on  mask(Single-port RAM){BlkNamePrefix='DelLine4', depth_bits=9, width_bits=5, dout_type=New data}
      mask prompts: BlkNamePrefix "Block name prefix:"; depth_bits "Address port width (2 to 16):"; width_bits "Data port width:"; dout_type "Output data during write:"
      mask help:
      | This block simulates a single-port RAM (based on hdllib).
      |
      | The address port width is limited to between 2 to 16 bits.
      mask init: same as FaceDet_x4/FaceDetection/DU/SplittedDL1/DelLine0_SPRAM_512x5
      mask StyleString: edit,edit,edit,popup(New data|Old data)
      mask Display: color('gray'); text(.5, .05, '{\fontsize{6}BRCM}', 'texmode', 'on', 'verticalAlignment', 'bottom', 'horizontalAlignment', 'center');
  DelLine5_SPRAM_512x5 : Subsystem  TreatAsAtomicUnit=on  mask(Single-port RAM){BlkNamePrefix='DelLine5', depth_bits=9, width_bits=5, dout_type=New data}
      mask prompts: BlkNamePrefix "Block name prefix:"; depth_bits "Address port width (2 to 16):"; width_bits "Data port width:"; dout_type "Output data during write:"
      mask help:
      | This block simulates a single-port RAM (based on hdllib).
      |
      | The address port width is limited to between 2 to 16 bits.
      mask init: same as FaceDet_x4/FaceDetection/DU/SplittedDL1/DelLine0_SPRAM_512x5
      mask StyleString: edit,edit,edit,popup(New data|Old data)
      mask Display: color('gray'); text(.5, .05, '{\fontsize{6}BRCM}', 'texmode', 'on', 'verticalAlignment', 'bottom', 'horizontalAlignment', 'center');
  DelLine6_SPRAM_512x5 : Subsystem  TreatAsAtomicUnit=on  mask(Single-port RAM){BlkNamePrefix='DelLine6', depth_bits=9, width_bits=5, dout_type=New data}
      mask prompts: BlkNamePrefix "Block name prefix:"; depth_bits "Address port width (2 to 16):"; width_bits "Data port width:"; dout_type "Output data during write:"
      mask help:
      | This block simulates a single-port RAM (based on hdllib).
      |
      | The address port width is limited to between 2 to 16 bits.
      mask init: same as FaceDet_x4/FaceDetection/DU/SplittedDL1/DelLine0_SPRAM_512x5
      mask StyleString: edit,edit,edit,popup(New data|Old data)
      mask Display: color('gray'); text(.5, .05, '{\fontsize{6}BRCM}', 'texmode', 'on', 'verticalAlignment', 'bottom', 'horizontalAlignment', 'center');
  DelLine7_SPRAM_512x5 : Subsystem  TreatAsAtomicUnit=on  mask(Single-port RAM){BlkNamePrefix='DelLine7', depth_bits=9, width_bits=5, dout_type=New data}
      mask prompts: BlkNamePrefix "Block name prefix:"; depth_bits "Address port width (2 to 16):"; width_bits "Data port width:"; dout_type "Output data during write:"
      mask help:
      | This block simulates a single-port RAM (based on hdllib).
      |
      | The address port width is limited to between 2 to 16 bits.
      mask init: same as FaceDet_x4/FaceDetection/DU/SplittedDL1/DelLine0_SPRAM_512x5
      mask StyleString: edit,edit,edit,popup(New data|Old data)
      mask Display: color('gray'); text(.5, .05, '{\fontsize{6}BRCM}', 'texmode', 'on', 'verticalAlignment', 'bottom', 'horizontalAlignment', 'center');
  GetAdr : simulink/Logic and Bit Operations/Extract Bits  SystemSampleTime=-1  bitsToExtract=Range of bits  numBits=8  bitIdxRange=[0 8]  outScalingMode=Treat bit field as an integer
  GetWrChunk : simulink/Logic and Bit Operations/Extract Bits  SystemSampleTime=-1  bitsToExtract=Range of bits  numBits=8  bitIdxRange=[9 11]  outScalingMode=Treat bit field as an integer
  LogicalOperator{0..7} (8 alike) : Logic  AllPortsSameDT=off  OutDataTypeStr=boolean
  DOut8x5 : Outport
  wires:
  CompareToConstant7/1 -> LogicalOperator7/1
  CompareToConstant6/1 -> LogicalOperator6/1
  CompareToConstant5/1 -> LogicalOperator5/1
  CompareToConstant4/1 -> LogicalOperator4/1
  CompareToConstant3/1 -> LogicalOperator3/1
  CompareToConstant2/1 -> LogicalOperator2/1
  CompareToConstant1/1 -> LogicalOperator1/1
  GetWrChunk/1 -> CompareToConstant7/1, CompareToConstant6/1, CompareToConstant5/1, CompareToConstant4/1, CompareToConstant3/1, CompareToConstant2/1, CompareToConstant1/1, CompareToConstant0/1
  CompareToConstant0/1 -> LogicalOperator0/1
  WrEn/1 -> LogicalOperator0/2, LogicalOperator1/2, LogicalOperator2/2, LogicalOperator3/2, LogicalOperator4/2, LogicalOperator5/2, LogicalOperator6/2, LogicalOperator7/2
  LogicalOperator7/1 -> DelLine7_SPRAM_512x5/3(we)
  LogicalOperator6/1 -> DelLine6_SPRAM_512x5/3(we)
  LogicalOperator5/1 -> DelLine5_SPRAM_512x5/3(we)
  LogicalOperator4/1 -> DelLine4_SPRAM_512x5/3(we)
  LogicalOperator3/1 -> DelLine3_SPRAM_512x5/3(we)
  DIn1x5/1 -> DelLine7_SPRAM_512x5/2(din), DelLine6_SPRAM_512x5/2(din), DelLine5_SPRAM_512x5/2(din), DelLine4_SPRAM_512x5/2(din), DelLine3_SPRAM_512x5/2(din), DelLine2_SPRAM_512x5/2(din), DelLine0_SPRAM_512x5/2(din), DelLine1_SPRAM_512x5/2(din)
  LogicalOperator2/1 -> DelLine2_SPRAM_512x5/3(we)
  LogicalOperator0/1 -> DelLine0_SPRAM_512x5/3(we)
  LogicalOperator1/1 -> DelLine1_SPRAM_512x5/3(we)
  WrAdr/1 -> GetWrChunk/1
  GetAdr/1 -> DelLine0_SPRAM_512x5/1(addr), DelLine2_SPRAM_512x5/1(addr), DelLine3_SPRAM_512x5/1(addr), DelLine4_SPRAM_512x5/1(addr), DelLine5_SPRAM_512x5/1(addr), DelLine7_SPRAM_512x5/1(addr), DelLine6_SPRAM_512x5/1(addr), DelLine1_SPRAM_512x5/1(addr)
  DataTypeConversion8/1 -> CombBus/8
  DataTypeConversion7/1 -> CombBus/7
  DataTypeConversion6/1 -> CombBus/6
  DataTypeConversion5/1 -> CombBus/5
  DataTypeConversion4/1 -> CombBus/4
  DataTypeConversion3/1 -> CombBus/3
  DataTypeConversion2/1 -> CombBus/2
  DataTypeConversion1/1 -> CombBus/1
  DelLine7_SPRAM_512x5/1(dout) -> DataTypeConversion8/1
  DelLine6_SPRAM_512x5/1(dout) -> DataTypeConversion7/1
  DelLine5_SPRAM_512x5/1(dout) -> DataTypeConversion6/1
  DelLine4_SPRAM_512x5/1(dout) -> DataTypeConversion5/1
  DelLine3_SPRAM_512x5/1(dout) -> DataTypeConversion4/1
  DelLine2_SPRAM_512x5/1(dout) -> DataTypeConversion3/1
  DelLine1_SPRAM_512x5/1(dout) -> DataTypeConversion2/1
  CombBus/1 -> DOut8x5/1
  RdAdr/1 -> GetAdr/1
  DelLine0_SPRAM_512x5/1(dout) -> DataTypeConversion1/1

== system FaceDet_x4/FaceDetection/FU/AccumulateAllFeatures ==
  note: AccumulatorBlock
  In : Inport
  En : Inport  Port=2
  Rst : Inport  Port=3
  Adder : Sum  OutDataTypeStr=uint(NBits)
  UDlyER : Subsystem  mask(Unit Delay Enabled Resettable){vinit=0, tsamp=-1}
      mask prompts: vinit "Initial condition:"; tsamp "Sample time:"
      mask help:
      | Normally, the output is the signal u delayed by one sample period.
      | When the reset signal R is true, the state is always set equal to the initial condition parameter.  This reset action is vectorized and supports scalar expansion.
      | When the enable signal is false, the block is disabled, and the state and output values do not change except for resets.  The enable action is vectorized and supports scalar expansion.
      mask Display: dpoly(1,[1 0],'z')
  Acc : Outport
  wires:
  En/1 -> UDlyER/2(E)
  Rst/1 -> UDlyER/3(R)
  In/1 -> Adder/1
  Adder/1 -> UDlyER/1(u), Acc/1
  UDlyER/1(y) -> Adder/2

== system FaceDet_x4/FaceDetection/FU/CalcIntegralImg ==
  DIn24x5 : Inport
  Rst : Inport  Port=2
  En : Inport  Port=3
  HorzRunningSum : Subsystem  RequirementInfo={} %GIDa_145c4b4e_900d_47e9_af66_464ac97b5d3c  TreatAsAtomicUnit=on
      mask Display: disp('Running Sum')
  TestValidNN : Subsystem  TreatAsAtomicUnit=on
  VerticalSum : Subsystem  TreatAsAtomicUnit=on
      mask Display: disp('Vertical Sum')
  MeanBlkVal : Outport
  ValidNN : Outport  Port=2
  DOut24x15 : Outport  Port=3
  wires:
  HorzRunningSum/1(DOut24x10) -> VerticalSum/1(DIn24x10)
  VerticalSum/2(MeanBlkVal) -> TestValidNN/1(MeanBlkVal), MeanBlkVal/1
  VerticalSum/1(DOut24x15) -> DOut24x15/1
  TestValidNN/1(ValidNN) -> ValidNN/1
  DIn24x5/1 -> HorzRunningSum/1(DIn24x5)
  En/1 -> HorzRunningSum/2(En)
  Rst/1 -> HorzRunningSum/3(Rst)

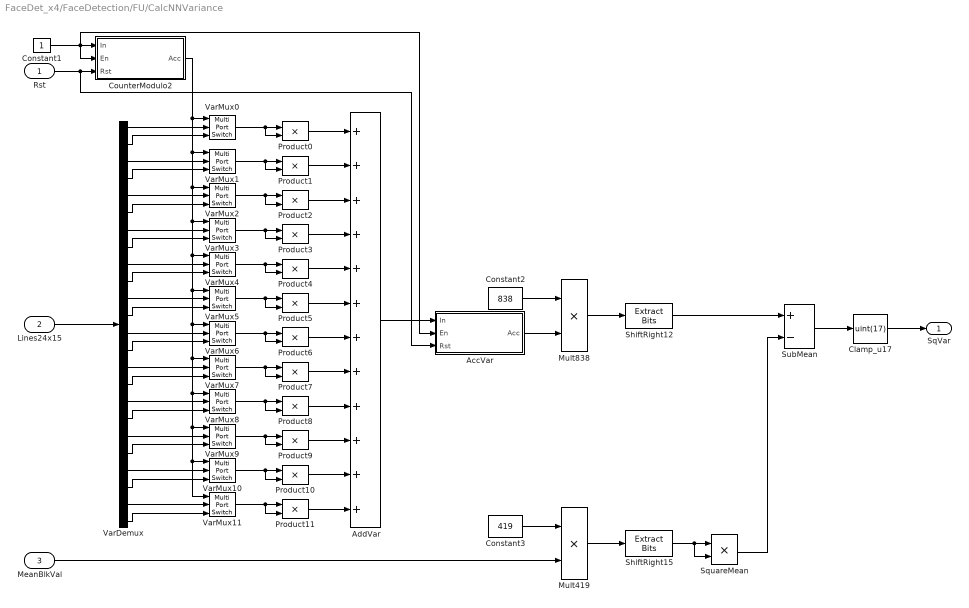
== system FaceDet_x4/FaceDetection/FU/CalcNNVariance ==
  Rst : Inport
  Lines24x15 : Inport  Port=2
  MeanBlkVal : Inport  Port=3
  AccVar : Subsystem  TreatAsAtomicUnit=on  mask(Accumulator){NBits=19}
      mask prompts: NBits "Number of Bits"
      mask help:
      | Accumulates incoming data. On reset only the state is initialized, meaning that when the reset is asserted the first valid output will be available from the next clock.
      | It is user responsiblity not to overcome the capacity of the accumulator.
      mask Help: web( ['E:\Ilia\Sightic\MakeVerilog\AccBlk\', 'AccBlkHelp.htm'] )
      mask Display: disp( 'Acc Blk\nBDelay = 0' )
  AddVar : Sum  Inputs=++++++++++++  OutDataTypeStr=uint(14)
  Clamp_u17 : DataTypeConversion  OutDataTypeStr=uint(17)  SaturateOnIntegerOverflow=on
  Constant1 : Constant  OutDataTypeStr=uint(1)
  Constant2 : Constant  Value=838  OutDataTypeStr=uint(10)
  Constant3 : Constant  Value=419  OutDataTypeStr=uint(9)
  CounterModulo2 : Subsystem  TreatAsAtomicUnit=on  mask(Accumulator){NBits=1}
      mask prompts: NBits "Number of Bits"
      mask help:
      | Accumulates incoming data. On reset only the state is initialized, meaning that when the reset is asserted the first valid output will be available from the next clock.
      | It is user responsiblity not to overcome the capacity of the accumulator.
      mask Help: web( ['E:\Ilia\Sightic\MakeVerilog\AccBlk\', 'AccBlkHelp.htm'] )
      mask Display: disp( 'Acc Blk\nBDelay = 0' )
  Mult419 : Product  OutDataTypeStr=uint(24)  RndMeth=Zero
  Mult838 : Product  OutDataTypeStr=uint(29)  RndMeth=Zero
  Product{0..11} (12 alike) : Product  OutDataTypeStr=uint(10)  RndMeth=Zero
  ShiftRight12 : simulink/Logic and Bit Operations/Extract Bits  SystemSampleTime=-1  bitsToExtract=Range of bits  numBits=8  bitIdxRange=[12 28]  outScalingMode=Treat bit field as an integer
  ShiftRight15 : simulink/Logic and Bit Operations/Extract Bits  SystemSampleTime=-1  bitsToExtract=Range of bits  numBits=8  bitIdxRange=[15 23]  outScalingMode=Treat bit field as an integer
  SquareMean : Product  OutDataTypeStr=uint(18)  RndMeth=Zero
  SubMean : Sum  Inputs=+-  OutDataTypeStr=sint(19)
  VarDemux : Demux  Outputs=24
  VarMux{0..11} (12 alike) : MultiPortSwitch  DataPortOrder=Zero-based contiguous  Inputs=2  zeroidx=on
  SqVar : Outport
  wires:
  Rst/1 -> CounterModulo2/3(Rst), AccVar/3(Rst)
  Constant1/1 -> CounterModulo2/1(In), CounterModulo2/2(En), AccVar/2(En)
  CounterModulo2/1(Acc) -> VarMux0/1, VarMux1/1, VarMux2/1, VarMux3/1, VarMux4/1, VarMux5/1, VarMux6/1, VarMux7/1, VarMux8/1, VarMux9/1, VarMux10/1, VarMux11/1
  VarMux0/1 -> Product0/1, Product0/2
  Product0/1 -> AddVar/1
  AddVar/1 -> AccVar/1(In)
  MeanBlkVal/1 -> Mult419/2
  SquareMean/1 -> SubMean/2
  SubMean/1 -> Clamp_u17/1
  Lines24x15/1 -> VarDemux/1
  VarDemux/1 -> VarMux0/2
  VarDemux/2 -> VarMux0/3
  VarDemux/3 -> VarMux1/2
  VarDemux/4 -> VarMux1/3
  VarDemux/5 -> VarMux2/2
  VarDemux/6 -> VarMux2/3
  VarDemux/7 -> VarMux3/2
  VarDemux/8 -> VarMux3/3
  VarDemux/9 -> VarMux4/2
  VarDemux/10 -> VarMux4/3
  VarDemux/11 -> VarMux5/2
  VarDemux/12 -> VarMux5/3
  VarDemux/13 -> VarMux6/2
  VarDemux/14 -> VarMux6/3
  VarDemux/15 -> VarMux7/2
  VarDemux/16 -> VarMux7/3
  VarDemux/17 -> VarMux8/2
  VarDemux/18 -> VarMux8/3
  VarDemux/19 -> VarMux9/2
  VarDemux/20 -> VarMux9/3
  VarDemux/21 -> VarMux10/2
  VarDemux/22 -> VarMux10/3
  VarDemux/23 -> VarMux11/2
  VarDemux/24 -> VarMux11/3
  VarMux1/1 -> Product1/2, Product1/1
  VarMux2/1 -> Product2/2, Product2/1
  VarMux3/1 -> Product3/2, Product3/1
  VarMux4/1 -> Product4/1, Product4/2
  VarMux5/1 -> Product5/1, Product5/2
  VarMux6/1 -> Product6/1, Product6/2
  VarMux7/1 -> Product7/1, Product7/2
  VarMux8/1 -> Product8/1, Product8/2
  VarMux9/1 -> Product9/1, Product9/2
  VarMux10/1 -> Product10/1, Product10/2
  VarMux11/1 -> Product11/1, Product11/2
  Product1/1 -> AddVar/2
  Product2/1 -> AddVar/3
  Product3/1 -> AddVar/4
  Product4/1 -> AddVar/5
  Product5/1 -> AddVar/6
  Product6/1 -> AddVar/7
  Product7/1 -> AddVar/8
  Product8/1 -> AddVar/9
  Product9/1 -> AddVar/10
  Product10/1 -> AddVar/11
  Product11/1 -> AddVar/12
  AccVar/1(Acc) -> Mult838/2
  Constant2/1 -> Mult838/1
  Mult838/1 -> ShiftRight12/1
  ShiftRight12/1 -> SubMean/1
  Constant3/1 -> Mult419/1
  Mult419/1 -> ShiftRight15/1
  ShiftRight15/1 -> SquareMean/1, SquareMean/2
  Clamp_u17/1 -> SqVar/1

== system FaceDet_x4/FaceDetection/FU/FeatureCalcMachine0 ==
  SqVar : Inport
  Lines24x15 : Inport  Port=2
  LineIdxs : Inport  Port=3
  NodeWeights : Inport  Port=4
  FeatureData : Inport  Port=5
  WeakTresh : Inport  Port=6
  CalcFeatureVal : Subsystem  TreatAsAtomicUnit=on
      mask Display: disp( 'BDly = \n\n' )
  CalcFeatureWeight : Subsystem  TreatAsAtomicUnit=on
  ExtractBits1 : simulink/Logic and Bit Operations/Extract Bits  SystemSampleTime=-1  bitsToExtract=Range of bits  numBits=8  bitIdxRange=[0 2]  outScalingMode=Treat bit field as an integer
  ExtractBits2 : simulink/Logic and Bit Operations/Extract Bits  SystemSampleTime=-1  bitsToExtract=Range of bits  numBits=8  bitIdxRange=[0 4]  outScalingMode=Treat bit field as an integer
  FinalFeatureWeight : Outport
  wires:
  ExtractBits1/1 -> CalcFeatureVal/3(NodeWeights)
  ExtractBits2/1 -> CalcFeatureVal/2(LineIdxs)
  SqVar/1 -> CalcFeatureWeight/2(SqVar)
  NodeWeights/1 -> ExtractBits1/1
  LineIdxs/1 -> ExtractBits2/1
  Lines24x15/1 -> CalcFeatureVal/1(Lines24x15)
  CalcFeatureVal/1(ColFeatureVal) -> CalcFeatureWeight/1(ColFeatureVal)
  FeatureData/1 -> CalcFeatureWeight/3(FeatureData)
  WeakTresh/1 -> CalcFeatureWeight/4(WeakTresh)
  CalcFeatureWeight/1(FinalFeatureWeight) -> FinalFeatureWeight/1

== system FaceDet_x4/FaceDetection/FU/FeatureCalcMachine1 ==
  SqVar : Inport
  Lines24x15 : Inport  Port=2
  LineIdxs : Inport  Port=3
  NodeWeights : Inport  Port=4
  FeatureData : Inport  Port=5
  WeakTresh : Inport  Port=6
  CalcFeatureVal : Subsystem  TreatAsAtomicUnit=on
      mask Display: disp( 'BDly = \n\n' )
  CalcFeatureWeight : Subsystem  TreatAsAtomicUnit=on
  ExtractBits1 : simulink/Logic and Bit Operations/Extract Bits  SystemSampleTime=-1  bitsToExtract=Range of bits  numBits=8  bitIdxRange=[3 5]  outScalingMode=Treat bit field as an integer
  ExtractBits2 : simulink/Logic and Bit Operations/Extract Bits  SystemSampleTime=-1  bitsToExtract=Range of bits  numBits=8  bitIdxRange=[5 9]  outScalingMode=Treat bit field as an integer
  FinalFeatureWeight : Outport
  wires:
  CalcFeatureWeight/1(FinalFeatureWeight) -> FinalFeatureWeight/1
  WeakTresh/1 -> CalcFeatureWeight/4(WeakTresh)
  FeatureData/1 -> CalcFeatureWeight/3(FeatureData)
  CalcFeatureVal/1(ColFeatureVal) -> CalcFeatureWeight/1(ColFeatureVal)
  Lines24x15/1 -> CalcFeatureVal/1(Lines24x15)
  LineIdxs/1 -> ExtractBits2/1
  NodeWeights/1 -> ExtractBits1/1
  SqVar/1 -> CalcFeatureWeight/2(SqVar)
  ExtractBits2/1 -> CalcFeatureVal/2(LineIdxs)
  ExtractBits1/1 -> CalcFeatureVal/3(NodeWeights)

== system FaceDet_x4/FaceDetection/FU/FeatureCalcMachine2 ==
  SqVar : Inport
  Lines24x15 : Inport  Port=2
  LineIdxs : Inport  Port=3
  NodeWeights : Inport  Port=4
  FeatureData : Inport  Port=5
  WeakTresh : Inport  Port=6
  CalcFeatureVal : Subsystem  TreatAsAtomicUnit=on
      mask Display: disp( 'BDly = \n\n' )
  CalcFeatureWeight : Subsystem  TreatAsAtomicUnit=on
  ExtractBits1 : simulink/Logic and Bit Operations/Extract Bits  SystemSampleTime=-1  bitsToExtract=Range of bits  numBits=8  bitIdxRange=[6 8]  outScalingMode=Treat bit field as an integer
  ExtractBits2 : simulink/Logic and Bit Operations/Extract Bits  SystemSampleTime=-1  bitsToExtract=Range of bits  numBits=8  bitIdxRange=[10 14]  outScalingMode=Treat bit field as an integer
  FinalFeatureWeight : Outport
  wires:
  ExtractBits1/1 -> CalcFeatureVal/3(NodeWeights)
  ExtractBits2/1 -> CalcFeatureVal/2(LineIdxs)
  SqVar/1 -> CalcFeatureWeight/2(SqVar)
  NodeWeights/1 -> ExtractBits1/1
  LineIdxs/1 -> ExtractBits2/1
  Lines24x15/1 -> CalcFeatureVal/1(Lines24x15)
  CalcFeatureVal/1(ColFeatureVal) -> CalcFeatureWeight/1(ColFeatureVal)
  FeatureData/1 -> CalcFeatureWeight/3(FeatureData)
  WeakTresh/1 -> CalcFeatureWeight/4(WeakTresh)
  CalcFeatureWeight/1(FinalFeatureWeight) -> FinalFeatureWeight/1

== system FaceDet_x4/FaceDetection/FU/FeatureCalcMachine3 ==
  SqVar : Inport
  Lines24x15 : Inport  Port=2
  LineIdxs : Inport  Port=3
  NodeWeights : Inport  Port=4
  FeatureData : Inport  Port=5
  WeakTresh : Inport  Port=6
  CalcFeatureVal : Subsystem  TreatAsAtomicUnit=on
      mask Display: disp( 'BDly = \n\n' )
  CalcFeatureWeight : Subsystem  TreatAsAtomicUnit=on
  ExtractBits1 : simulink/Logic and Bit Operations/Extract Bits  SystemSampleTime=-1  bitsToExtract=Range of bits  numBits=8  bitIdxRange=[9 11]  outScalingMode=Treat bit field as an integer
  ExtractBits2 : simulink/Logic and Bit Operations/Extract Bits  SystemSampleTime=-1  bitsToExtract=Range of bits  numBits=8  bitIdxRange=[15 19]  outScalingMode=Treat bit field as an integer
  FinalFeatureWeight : Outport
  wires:
  CalcFeatureWeight/1(FinalFeatureWeight) -> FinalFeatureWeight/1
  WeakTresh/1 -> CalcFeatureWeight/4(WeakTresh)
  FeatureData/1 -> CalcFeatureWeight/3(FeatureData)
  CalcFeatureVal/1(ColFeatureVal) -> CalcFeatureWeight/1(ColFeatureVal)
  Lines24x15/1 -> CalcFeatureVal/1(Lines24x15)
  LineIdxs/1 -> ExtractBits2/1
  NodeWeights/1 -> ExtractBits1/1
  SqVar/1 -> CalcFeatureWeight/2(SqVar)
  ExtractBits2/1 -> CalcFeatureVal/2(LineIdxs)
  ExtractBits1/1 -> CalcFeatureVal/3(NodeWeights)
